simulink model "microgrid_mpc3"  (R2025a)
settings: Solver=FixedStepAuto  StartTime=0.0  StopTime=0.2  FixedStep=Ts  RelTol=1e-3
values from neighbouring files (symbols this model uses):
  C = Kpcc*[0 alpha R]    [parametros_micro.m]
  D = min(max(D,0),1)    [VSI_PWM.m]    (also in VSI_PWM_Modulator.m; der_delay_mpc.m = 0.0005; der_mpc.m = 0.0005; parametros_micro.m = [0 1])
  L = 5e-3    (= 0.005)    [der.m]    (also in der_delay.m; der_delay_mpc.m; der_mpc.m; der_mpc_acoplado.m)
  plant = c2d(plant_c,Ts)    [parametros_micro.m]
  R = 0.1    [der.m]    (also in der_delay.m; der_delay_mpc.m; der_mpc.m; der_mpc_acoplado.m)
  Ts = 1e-5    (= 1e-05)    [der_delay_mpc.m]    (also in der_mpc.m; der_mpc_acoplado.m; parametros_micro.m = 5e-05; parametros_micro2.m = 5e-05)
  Vdc = 400    [parametros_micro.m]    (also in parametros_micro2.m)
libraries: eeRmsMeasurement x4, mpclib x3, eeStairGenerator x1
settings Model: Creator=Acer  LastModifiedBy=cmparedesv
settings SolverCC: AlgebraicLoopSolver=TrustRegion
settings DebuggingCC: UnconnectedInputMsg=warning  UnconnectedOutputMsg=warning  UnconnectedLineMsg=warning
settings ModelReferenceCC: EnableRefExpFcnMdlSchedulingChecks=on
settings RTWCC: GPUComputeCapability=3.5  DLArmComputeVersion=19.05

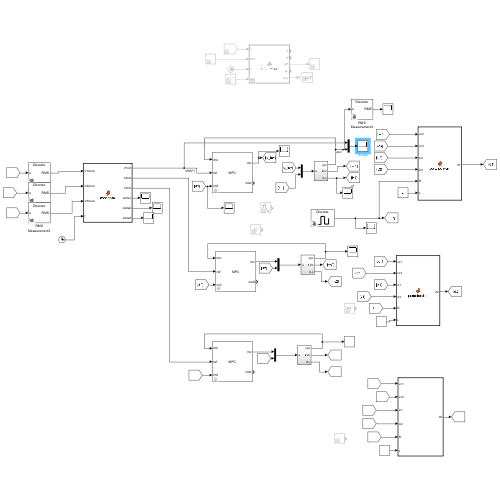
[thumbnail: Simulink's stored preview of the top-level diagram]
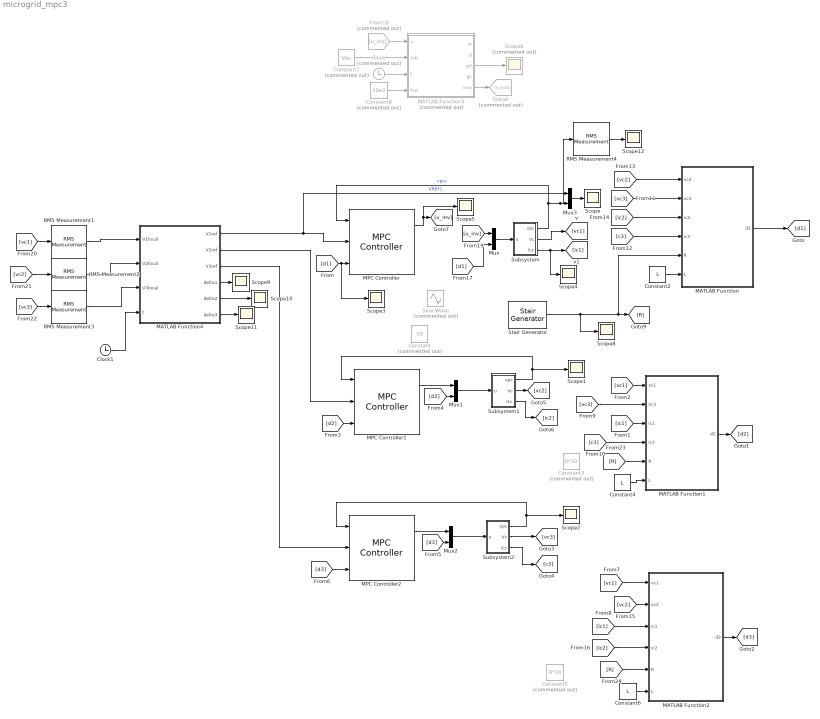
== system microgrid_mpc3 ==
  Clock : Clock  Commented=on
  Clock1 : Clock
  Constant : Constant  Commented=on  Value=10
  Constant2 : Constant  Value=L
  Constant3 : Constant  Commented=on  Value=R*30
  Constant4 : Constant  Value=L
  Constant5 : Constant  Commented=on  Value=R*30
  Constant6 : Constant  Value=L
  Constant7 : Constant  Commented=on  Value=Vdc
  Constant8 : Constant  Commented=on  Value=10e3
  From18 : From  Commented=on  GotoTag=u_inv
  Goto8 : Goto  Commented=on  GotoTag=v_inv1
  MATLAB Function : MATLAB Function  TreatAsAtomicUnit=on
  MATLAB Function1 : MATLAB Function  TreatAsAtomicUnit=on
  MATLAB Function2 : MATLAB Function  TreatAsAtomicUnit=on
  MATLAB Function3 : MATLAB Function  Commented=on  TreatAsAtomicUnit=on
  MATLAB Function4 : MATLAB Function  TreatAsAtomicUnit=on
  MPC Controller : mpclib/MPC Controller  SCDEnableBlockLinearizationSpecification=on  mpcobj=mpcobj  is_multiple=0  enable_value=0  return_u0=off  updateMPCinCallerWorkspace=on  md_inport=on  mv_inport=off  uref_inport=off  return_cost=on  return_mvseq=off  return_qpstatus=off  return_xseq=off  return_state=off  return_ovseq=off  state_inport=off  umin_inport=off  umax_inport=off  ymin_inport=off  ymax_inport=off  cc_inport=off  ywt_inport=off  uwt_inport=off  duwt_inport=off  rhoeps_inport=off  pm_inport=off  MaximumP=10  HorizonChoice=FixedHorizon  n_ts=5e-05  n_p=20  n_mv=1  n_md=1  n_ud=0  n_mo=1  n_uo=0  BlockDataType=double  SampleTimeInherited=off  switch_inport=off
  MPC Controller1 : mpclib/MPC Controller  SCDEnableBlockLinearizationSpecification=on  mpcobj=mpcobj  is_multiple=0  enable_value=0  return_u0=off  updateMPCinCallerWorkspace=on  md_inport=on  mv_inport=off  uref_inport=off  return_cost=on  return_mvseq=off  return_qpstatus=off  return_xseq=off  return_state=off  return_ovseq=off  state_inport=off  umin_inport=off  umax_inport=off  ymin_inport=off  ymax_inport=off  cc_inport=off  ywt_inport=off  uwt_inport=off  duwt_inport=off  rhoeps_inport=off  pm_inport=off  MaximumP=10  HorizonChoice=FixedHorizon  n_ts=5e-05  n_p=20  n_mv=1  n_md=1  n_ud=0  n_mo=1  n_uo=0  BlockDataType=double  SampleTimeInherited=off  switch_inport=off
  MPC Controller2 : mpclib/MPC Controller  SCDEnableBlockLinearizationSpecification=on  mpcobj=mpcobj  is_multiple=0  enable_value=0  return_u0=off  updateMPCinCallerWorkspace=on  md_inport=on  mv_inport=off  uref_inport=off  return_cost=on  return_mvseq=off  return_qpstatus=off  return_xseq=off  return_state=off  return_ovseq=off  state_inport=off  umin_inport=off  umax_inport=off  ymin_inport=off  ymax_inport=off  cc_inport=off  ywt_inport=off  uwt_inport=off  duwt_inport=off  rhoeps_inport=off  pm_inport=off  MaximumP=10  HorizonChoice=FixedHorizon  n_ts=5e-05  n_p=20  n_mv=1  n_md=1  n_ud=0  n_mo=1  n_uo=0  BlockDataType=double  SampleTimeInherited=off  switch_inport=off
  Mux{,1..3} (4 alike) : Mux  Inputs=2
  RMS Measurement{1..4} (4 alike) : eeRmsMeasurement/RMS Measurement  LabelModeActiveChoice=Total  F=60  SpecifyHarmonics=off  K=[0 1 2]  Ts=Ts
  Scope{,1..5,8..12} (11 alike) : Scope
      Scope settings: ActiveDisplayYMinimum=-221.47313854310383  ActiveDisplayYMaximum=221.36211600333627
      Scope1 settings: ActiveDisplayYMinimum=-213.42062  ActiveDisplayYMaximum=219.50862
      Scope10 settings: ActiveDisplayYMinimum=-0.63291  ActiveDisplayYMaximum=5.99623  DataLoggingVariableName=ScopeData10
      Scope11 settings: ActiveDisplayYMinimum=-0.63291  ActiveDisplayYMaximum=5.99623  DataLoggingVariableName=ScopeData11
      Scope12 settings: ActiveDisplayYMinimum=-15.27318  ActiveDisplayYMaximum=137.45859  DataLoggingVariableName=ScopeData12
      Scope2 settings: ActiveDisplayYMinimum=-213.42062  ActiveDisplayYMaximum=219.50862  DataLoggingVariableName=ScopeData2
      Scope3 settings: ActiveDisplayYMinimum=-37.60883  ActiveDisplayYMaximum=64.36422  DataLoggingVariableName=ScopeData3
      Scope4 settings: ActiveDisplayYMinimum=-33.39286  ActiveDisplayYMaximum=38.63484  DataLoggingVariableName=ScopeData4
      Scope5 settings: ActiveDisplayYMinimum=-250  ActiveDisplayYMaximum=250  DataLoggingVariableName=ScopeData5
      Scope8 settings: ActiveDisplayYMinimum=-2.625  ActiveDisplayYMaximum=33.625  DataLoggingVariableName=ScopeData8
      Scope9 settings: ActiveDisplayYMinimum=-0.63291  ActiveDisplayYMaximum=5.99623  DataLoggingVariableName=ScopeData9
  Scope6 : Scope  Commented=on
      settings: ActiveDisplayYMinimum=-0.125  ActiveDisplayYMaximum=1.125  DataLoggingVariableName=ScopeData6
  Sine Wave : Sin  Commented=on  Amplitude=120*sqrt(2)  Frequency=2*pi*60  SampleTime=Ts
  Stair Generator : eeStairGenerator/Stair Generator  LabelModeActiveChoice=Discrete  TimeInput=[0 .05 .1 0.15]  AmplitudeInput=[R 30*R 2*R 22*R]  SampleTime=Ts  RepeatPattern=off  OutDataTypeStr=double
  Subsystem : Subsystem
  Subsystem1 : Subsystem
  Subsystem2 : Subsystem
  wires:
  Subsystem/1(vpc) -> RMS Measurement4/1, Mux3/2, MPC Controller/1  "vpcc"
  MPC Controller/1 -> [u_inv], Scope5/1
  Mux/1 -> Subsystem/1(u)
  Constant2/1 -> MATLAB Function/6(L)
  Subsystem1/1(vpc) -> MPC Controller1/1, Scope1/1
  Constant4/1 -> MATLAB Function1/6(L)
  MPC Controller1/1 -> Mux1/1
  Mux1/1 -> Subsystem1/1(u)
  Subsystem2/1(vpc) -> MPC Controller2/1, Scope2/1
  Constant6/1 -> MATLAB Function2/6(L)
  MPC Controller2/1 -> Mux2/1
  Mux2/1 -> Subsystem2/1(u)
  MATLAB Function/1(d1) -> [d1]
  [d1] -> Scope3/1, MPC Controller/3
  Subsystem/2(Vc) -> [vc1]
  Subsystem/3(ILc) -> Scope4/1, [ic1]
  [vc1] -> MATLAB Function1/1(vc1)
  [ic1] -> MATLAB Function1/3(ic1)
  MATLAB Function1/1(d2) -> [d2]
  [d2] -> MPC Controller1/3
  [d2] -> Mux1/2
  [d3] -> Mux2/2
  MATLAB Function2/1(d3) -> [d3]
  [d3] -> MPC Controller2/3
  [vc1] -> MATLAB Function2/1(vc1)
  [ic1] -> MATLAB Function2/3(ic1)
  Subsystem2/2(Vc) -> [vc3]
  Subsystem2/3(ILc) -> [c3]
  [vc3] -> MATLAB Function1/2(vc3)
  [c3] -> MATLAB Function1/4(ic3)
  [vc3] -> MATLAB Function/2(vc3)
  [c3] -> MATLAB Function/4(ic3)
  Subsystem1/2(Vc) -> [vc2]
  Subsystem1/3(ILc) -> [ic2]
  [vc2] -> MATLAB Function/1(vc2)
  [ic2] -> MATLAB Function/3(ic2)
  [ic2] -> MATLAB Function2/4(ic2)
  [vc2] -> MATLAB Function2/2(vc2)
  [d1] -> Mux/2
  Mux3/1 -> Scope/1
  From18/1 -> MATLAB Function3/1(u)
  Constant7/1 -> MATLAB Function3/2(Vdc)
  Constant8/1 -> MATLAB Function3/4(fsw)
  MATLAB Function3/5(vInv) -> Goto8/1
  [u_inv] -> Mux/1
  Clock/1 -> MATLAB Function3/3(t)
  MATLAB Function3/3(gH) -> Scope6/1
  [vc2] -> RMS Measurement2/1
  MATLAB Function4/1(V1ref) -> Mux3/1, MPC Controller/2  "VREF1"
  MATLAB Function4/2(V2ref) -> MPC Controller1/2
  MATLAB Function4/3(V3ref) -> MPC Controller2/2
  [vc1] -> RMS Measurement1/1
  RMS Measurement1/1 -> MATLAB Function4/1(V1local)
  RMS Measurement2/1 -> MATLAB Function4/2(V2local)
  [vc3] -> RMS Measurement3/1
  RMS Measurement3/1 -> MATLAB Function4/3(V3local)
  Clock1/1 -> MATLAB Function4/4(t)
  [R] -> MATLAB Function2/5(R)
  Stair Generator/1 -> Scope8/1, [R], MATLAB Function/5(R)
  [R] -> MATLAB Function1/5(R)
  MATLAB Function4/4(delta1) -> Scope9/1
  MATLAB Function4/5(delta2) -> Scope10/1
  MATLAB Function4/6(delta3) -> Scope11/1
  RMS Measurement4/1 -> Scope12/1

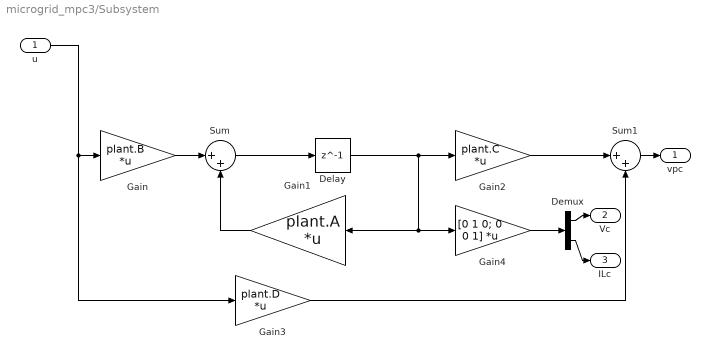
== system microgrid_mpc3/Subsystem ==
  u : Inport
  Delay : Delay  DelayLength=1  SampleTime=Ts
  Demux : Demux  Outputs=2
  Gain : Gain  Gain=plant.B  Multiplication=Matrix(K*u)
  Gain1 : Gain  Gain=plant.A  Multiplication=Matrix(K*u)
  Gain2 : Gain  Gain=plant.C  Multiplication=Matrix(K*u)
  Gain3 : Gain  Gain=plant.D  Multiplication=Matrix(K*u)
  Gain4 : Gain  Gain=[0 1 0; 0 0 1]  Multiplication=Matrix(K*u)
  Sum : Sum  Inputs=|++
  Sum1 : Sum  Inputs=|++
  vpc : Outport
  Vc : Outport  Port=2
  ILc : Outport  Port=3
  wires:
  Delay/1 -> Gain4/1, Gain1/1, Gain2/1
  Gain4/1 -> Demux/1
  Gain3/1 -> Sum1/2
  Sum/1 -> Delay/1
  Gain2/1 -> Sum1/1
  Gain1/1 -> Sum/2
  u/1 -> Gain3/1, Gain/1
  Demux/1 -> Vc/1
  Gain/1 -> Sum/1
  Sum1/1 -> vpc/1
  Demux/2 -> ILc/1

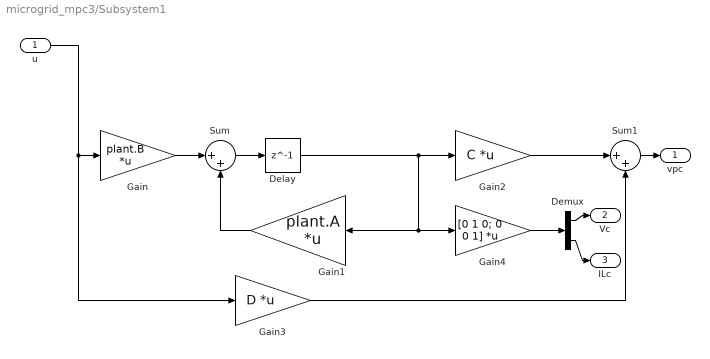
== system microgrid_mpc3/Subsystem1 ==
  u : Inport
  Delay : Delay  DelayLength=1  SampleTime=Ts
  Demux : Demux  Outputs=2
  Gain : Gain  Gain=plant.B  Multiplication=Matrix(K*u)
  Gain1 : Gain  Gain=plant.A  Multiplication=Matrix(K*u)
  Gain2 : Gain  Gain=C  Multiplication=Matrix(K*u)
  Gain3 : Gain  Gain=D  Multiplication=Matrix(K*u)
  Gain4 : Gain  Gain=[0 1 0; 0 0 1]  Multiplication=Matrix(K*u)
  Sum : Sum  Inputs=|++
  Sum1 : Sum  Inputs=|++
  vpc : Outport
  Vc : Outport  Port=2
  ILc : Outport  Port=3
  wires:
  Delay/1 -> Gain4/1, Gain1/1, Gain2/1
  Gain4/1 -> Demux/1
  Gain3/1 -> Sum1/2
  Sum/1 -> Delay/1
  Gain2/1 -> Sum1/1
  Gain1/1 -> Sum/2
  u/1 -> Gain3/1, Gain/1
  Demux/1 -> Vc/1
  Gain/1 -> Sum/1
  Sum1/1 -> vpc/1
  Demux/2 -> ILc/1

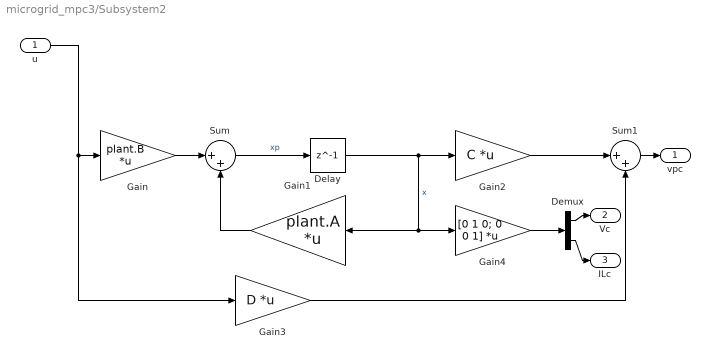
== system microgrid_mpc3/Subsystem2 ==
  u : Inport
  Delay : Delay  DelayLength=1  SampleTime=Ts
  Demux : Demux  Outputs=2
  Gain : Gain  Gain=plant.B  Multiplication=Matrix(K*u)
  Gain1 : Gain  Gain=plant.A  Multiplication=Matrix(K*u)
  Gain2 : Gain  Gain=C  Multiplication=Matrix(K*u)
  Gain3 : Gain  Gain=D  Multiplication=Matrix(K*u)
  Gain4 : Gain  Gain=[0 1 0; 0 0 1]  Multiplication=Matrix(K*u)
  Sum : Sum  Inputs=|++
  Sum1 : Sum  Inputs=|++
  vpc : Outport
  Vc : Outport  Port=2
  ILc : Outport  Port=3
  wires:
  Delay/1 -> Gain4/1, Gain1/1, Gain2/1  "x"
  Gain4/1 -> Demux/1
  Gain3/1 -> Sum1/2
  Sum/1 -> Delay/1  "xp"
  Gain2/1 -> Sum1/1
  Gain1/1 -> Sum/2
  u/1 -> Gain3/1, Gain/1
  Demux/1 -> Vc/1
  Gain/1 -> Sum/1
  Sum1/1 -> vpc/1
  Demux/2 -> ILc/1

== matlab function microgrid_mpc3/MATLAB Function1 ==
  data: vc1 input; d2 output; vc3 input; ic1 input; ic3 input; R input; L input
function d2 = perturbacion(vc1,vc3,ic1,ic3,R,L)
Lc = .5e-3;
alpha = L/Lc;

K = 1/(1 + 3*alpha);

d2=K*(alpha*(vc1+vc3)+R*(ic1+ic3));

== matlab function microgrid_mpc3/MATLAB Function ==
  data: vc2 input; d1 output; vc3 input; ic2 input; ic3 input; R input; L input
function d1 = perturbacion(vc2,vc3,ic2,ic3,R,L)
Lc = .5e-3;
alpha = L/Lc;

K = 1/(1 + 3*alpha);

d1=K*(alpha*(vc2+vc3)+R*(ic2+ic3));

== matlab function microgrid_mpc3/MATLAB Function2 ==
  data: vc1 input; vc2 input; ic1 input; d3 output; ic2 input; R input; L input
function d3 = perturbacion(vc1,vc2,ic1,ic2,R,L)
Lc = .5e-3;
alpha = L/Lc;

K = 1/(1 + 3*alpha);

d3=K*(alpha*(vc2+vc1)+R*(ic2+ic1));

== matlab function microgrid_mpc3/MATLAB Function3 ==
  data: u input; m output; Vdc input; t input; fsw input; D output; gH output; gL output; vInv output
function [m,D,gH,gL,vInv] = VSI_PWM(u,Vdc,t,fsw)
% VSI_PWM
% Genera PWM bipolar para un VSI monofasico de dos niveles.
%
% Entradas:
%   u   = referencia de voltaje del MPC [V]
%   Vdc = tension del bus DC [V]
%   t   = tiempo actual de simulacion [s]
%   fsw = frecuencia de conmutacion [Hz]
%
% Salidas:
%   m    = indice de modulacion [-1,1]
%   D    = duty cycle [0,1]
%   gH   = gate del interruptor superior
%   gL   = gate complementario
%   vInv = tension instantanea ideal del VSI [V]
%
% Modelo PWM bipolar:
%   m = 2*u/Vdc
%   D = (1+m)/2
%
% Portadora triangular:
%   carrier = 1 - 4*abs(frac(t*fsw)-0.5)
%
% Conmutacion:
%   gH = 1 si m >= carrier
%   gL = 1 - gH
%
% Tension de salida:
%   vInv = Vdc*(2*gH-1)
%
% NOTA:
% Este modelo no incluye tiempo muerto. Para una implementacion
% de potencia mas detallada, debe incorporarse dead-time entre
% gH y gL.

% Proteccion contra valores invalidos
if Vdc <= 0 || fsw <= 0
    m = 0;
    D = 0.5;
    gH = 0;
    gL = 0;
    vInv = 0;
    return;
end

% ------------------------------------------------------------
% 1. Indice de modulacion generado por el MPC
% ------------------------------------------------------------
m = 2*u/Vdc;

% Saturacion del indice de modulacion
m = min(max(m,-1),1);

% ------------------------------------------------------------
% 2. Duty cycle equivalente
% ------------------------------------------------------------
D = (1+m)/2;
D = min(max(D,0),1);

% ------------------------------------------------------------
% 3. Portadora triangular normalizada [-1,1]
% ------------------------------------------------------------
phase = t*fsw - floor(t*fsw);
carrier = 1 - 4*abs(phase - 0.5);

% ------------------------------------------------------------
% 4. Generacion de PWM
% ------------------------------------------------------------
if m >= carrier
    gH = 1;
else
    gH = 0;
end

% Interruptor complementario
gL = 1 - gH;

% ------------------------------------------------------------
% 5. Tension instantanea del VSI
% ------------------------------------------------------------
vInv = Vdc*(2*gH - 1);

end

== matlab function microgrid_mpc3/MATLAB Function4 ==
  data: V1local input; V1ref output; V2local input; V3local input; V2ref output; V3ref output; delta1 output; delta2 output; delta3 output; t input
function [V1ref,V2ref,V3ref,delta1,delta2,delta3] = ...
    consenso(V1local,V2local,V3local,t)
% ================================================================
% CONTROL SECUNDARIO DISTRIBUIDO - CONSENSO
%
% Topologia de comunicacion:
%
%       VSI 1 <------> VSI 2 <------> VSI 3
%
% Matriz de adyacencia:
%
%       Ag = [0 1 0
%             1 0 1
%             0 1 0]
%
% Matriz Laplaciana:
%
%       L = [ 1 -1  0
%            -1  2 -1
%             0 -1  1]
%
% Ley de control:
%
%       delta_dot = kI*e - kc*L*delta
%
% ================================================================


% ================================================================
% CONTROL SECUNDARIO DISTRIBUIDO POR CONSENSO
% Tres VSI conectados en paralelo
%
% Objetivo:
%       V_i --> 120 Vrms
%       delta_1 = delta_2 = delta_3
%
% El consenso NO genera directamente la tension del inversor.
% Genera una correccion secundaria delta_i que modifica la
% referencia de amplitud del MPC.
%
% ---------------------------------------------------------------
% REFERENCIA DE TENSION
%
%       V_i^ref = V_nom + delta_i
%
% donde:
%       V_nom = 120 Vrms
%
% La referencia sinusoidal que recibe cada MPC es:
%
%       r_i(t) = sqrt(2)*V_i^ref*sin(2*pi*f*t)
%
% ---------------------------------------------------------------
% ERROR LOCAL DE TENSION
%
%       e_i = V_nom - V_i_local
%
% ---------------------------------------------------------------
% LEY DE CONSENSO
%
% Para un grafo completo de 3 inversores:
%
%       delta_dot_1 =
%           kI*e_1 + kc[(delta_2-delta_1)+(delta_3-delta_1)]
%
%       delta_dot_2 =
%           kI*e_2 + kc[(delta_1-delta_2)+(delta_3-delta_2)]
%
%       delta_dot_3 =
%           kI*e_3 + kc[(delta_1-delta_3)+(delta_2-delta_3)]
%
% En forma matricial:
%
%       delta_dot = kI*e - kc*L*delta
%
% donde:
%
%       delta = [delta_1 delta_2 delta_3]'
%
%       e = [e_1 e_2 e_3]'
%
%       L = [ 2 -1 -1
%            -1  2 -1
%            -1 -1  2 ]
%
% es el Laplaciano del grafo de comunicacion.
%
% ---------------------------------------------------------------
% DISCRETIZACION
%
% Como Ts = 50 us:
%
%       delta_i(k+1) =
%           delta_i(k) + Ts*delta_dot_i(k)
%
% ---------------------------------------------------------------
% SALIDA
%
%       V_i^ref = 120 + delta_i
%
% Estas referencias entran posteriormente a los tres MPC.
% ================================================================


% ---------------- PARAMETROS ----------------

Ts = 50e-6;          % Tiempo de muestreo [s]

Vnom = 120;          % Tension nominal [Vrms]

f = 60;              % Frecuencia de referencia [Hz]

% Ganancia integral del error de tension
kI = 5;

% Ganancia de consenso
kc = 10;

% Limites de la correccion secundaria
delta_min = -10;     % [V]
delta_max =  10;     % [V]


% ---------------- ESTADOS DEL CONSENSO ----------------

% delta_i son los estados del controlador secundario.
%
% Se conservan entre llamadas mediante "persistent".

persistent delta_1 delta_2 delta_3

if isempty(delta_1)

    delta_1 = 0;
    delta_2 = 0;
    delta_3 = 0;

end


% ================================================================
% 1. ERROR LOCAL DE TENSION
% ================================================================

% Formalmente:
%
%       e_i = V_nom - V_i_local

e_1 = Vnom - V1local;
e_2 = Vnom - V2local;
e_3 = Vnom - V3local;


% ================================================================
% 2. TERMINO DE CONSENSO
% ================================================================
% ================================================================
% 2. MATRIZ DE ADYACENCIA
% ================================================================
% Ag = [0 1 1;
%       1 0 1;
%       1 1 0]; %todos los inversores comparten comunicacion
% 

Ag = [0 1 0;
      1 0 1;
      0 1 0];


% ================================================================
% 3. MATRIZ DE GRADOS
% ================================================================

Dg = [1 0 0;
      0 2 0;
      0 0 1];

% Dg = [2 0 0;
%       0 2 0;
%       0 0 2]; %todos comparten


% ================================================================
% 4. MATRIZ LAPLACIANA
% ================================================================

L = Dg - Ag;


% ================================================================
% 5. VECTOR DE CORRECCIONES
% ================================================================
delta = [delta_1;
         delta_2;
         delta_3];
% Cada inversor compara su correccion con las correcciones de
% sus vecinos.
% deltap = kI*e-kc*L*delta
% Para el grafo completo: (todas las conexion)
%
%       c_1 = (delta_2-delta_1)+(delta_3-delta_1)
%
%       c_2 = (delta_1-delta_2)+(delta_3-delta_2)
%
%       c_3 = (delta_1-delta_3)+(delta_2-delta_3)

%c_1 = (delta_2-delta_1) + (delta_3-delta_1);

%c_2 = (delta_1-delta_2) + (delta_3-delta_2);

%c_3 = (delta_1-delta_3) + (delta_2-delta_3);

% ================================================================
% 6. VECTOR DE ERRORES
% ================================================================

e = [e_1;
     e_2;
     e_3];

% ================================================================
% 7. LEY DE CONSENSO
%
%       delta_dot = kI*e - kc*L*delta
% ================================================================

delta_dot = kI*e - kc*L*delta;


% ================================================================
% 8. DISCRETIZACION metodo de euler
%
%       delta(k+1) =
%       delta(k) + Ts*delta_dot(k)
% ================================================================

delta = delta + Ts*delta_dot;

% ================================================================
% 5. SATURACION DE LA CORRECCION
% ================================================================

delta_1 = min(max(delta(1),delta_min),delta_max);

delta_2 = min(max(delta(2),delta_min),delta_max);

delta_3 = min(max(delta(3),delta_min),delta_max);


% ================================================================
% 6. REFERENCIA DE AMPLITUD PARA CADA MPC
% ================================================================

%       V_i^ref = V_nom + delta_i

V1ref = Vnom + delta_1;

V2ref = Vnom + delta_2;

V3ref = Vnom + delta_3;

V1ref=sqrt(2)*V1ref*sin(2*pi*f*t);
V2ref=sqrt(2)*V2ref*sin(2*pi*f*t);
V3ref=sqrt(2)*V3ref*sin(2*pi*f*t);


% ================================================================
% 7. SALIDA DE LAS VARIABLES INTERNAS
% ================================================================

delta1 = delta_1;

delta2 = delta_2;

delta3 = delta_3;

end
